simulink model "obsmod_mdl"  (R2021b)
settings: Solver=ode1  StartTime=0.0  StopTime=10  FixedStep=0.001  MaxStep=0.25  MinStep=0.01  RelTol=1e-3  EnableMultiTasking=on
values from neighbouring files (symbols this model uses):
  A = [0 1; 0 0]    [pendulum_data.m]
  Am = A+B*Lx    [obsmod_data.m]    (also in outmod_data.m; outmodc_data.m; stmod_data.m = A+B*F)
  B = [0;1]    [pendulum_data.m]
  Bm = B*-inv(Cm*inv(Am)*B)    [obsmod_data.m]    (also in outmod_data.m; outmodc_data.m; stmod_data.m = B*G)
  C = C([1,3],:)    [comp_data.m]    (also in pendulum_data.m = [1 1])
  G = -inv(C*inv(A+B*F)*B)    [obsint_data.m]    (also in stmod_data.m = -inv(H*inv(A+B*F)*B))
  L = -inv(S*B)*(S*Am-Phi*S)    [stmod_data.m]
  rho = 1    [comp_data.m]    (also in obsint_data.m; obsmod_data.m; outmod_data.m; outmodc_data.m)
  S = rpp(A,B,psm)    [obsint_data.m]    (also in stint_data.m = rpp(A,B,sp); stmod_data.m = inv(S*B)*S; streg_data.m = rpp(A,B,sp))
  x0 = zeros(1,n)    [comp_data.m]    (also in obsint_data.m; obsmod_data.m; outmod_data.m; outmodc_data.m)
  z0 = zeros(1,n)    [obsint_data.m]    (also in obsmod_data.m; pendulum_data.m)
undefined symbols (not defined in the file or in its folder): F, Lr, Lx, m, n, P
settings Model: Creator=w.schwamm  LastModifiedBy=w.schwamm
settings SolverCC: AlgebraicLoopSolver=TrustRegion
settings DataIOCC: SaveOutput=off  SaveTime=off  ReturnWorkspaceOutputs=off  StateSaveName=x  TimeSaveName=t  OutputSaveName=y
settings OptimizationCC: LifeSpan=inf
settings DebuggingCC: SFUnexpectedBacktrackingDiag=warning  SFNoUnconditionalDefaultTransitionDiag=warning  SFMachineParentedDataDiag=warning  ArithmeticOperatorsInVariantConditions=warning
settings SFSimCC: SimUseLocalCustomCode=off  CustomCodeUndefinedFunction=UseInterfaceOnly
settings RTWCC: RTWUseLocalCustomCode=off
settings CodeAppCC: StateflowObjectComments=on
settings GRTTargetCC: TargetLangStandard=C89/C90 (ANSI)
settings ConfigComp: CovMetricSettings=dw  CovSaveCumulativeToWorkspaceVar=on  CovSaveSingleToWorkspaceVar=on  CovExternalEMLEnable=off

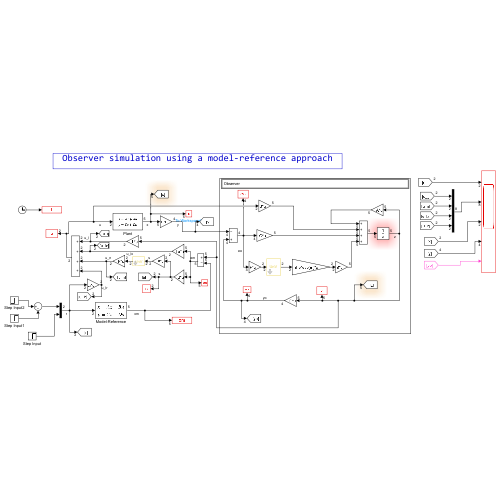
[thumbnail: Simulink's stored preview of the top-level diagram]
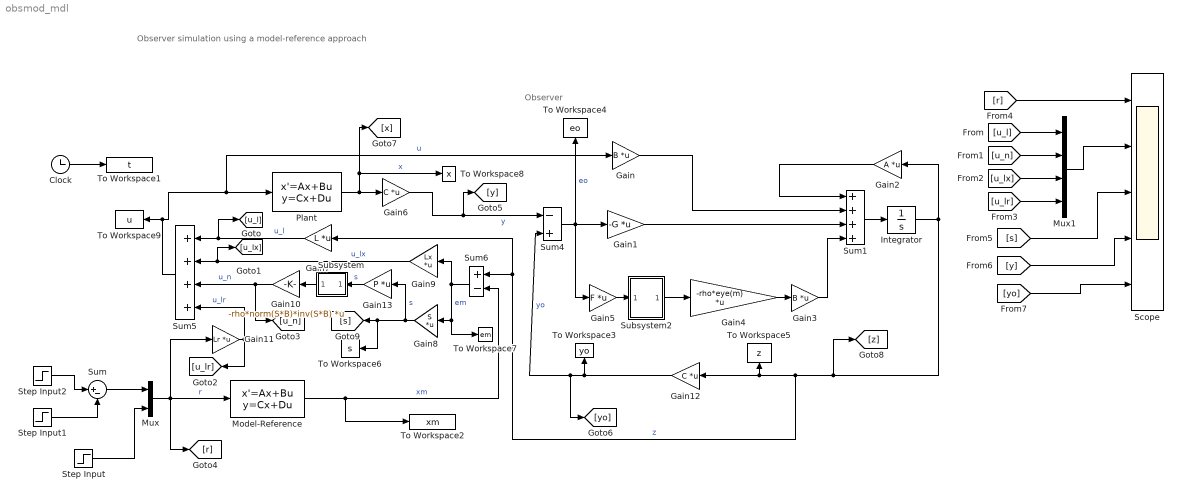
== system obsmod_mdl ==
  note: Observer
  note: Observer simulation using a model-reference approach
  Clock : Clock
  Gain : Gain  Gain=B  Multiplication=Matrix(K*u)
  Gain1 : Gain  Gain=-G  Multiplication=Matrix(K*u)
  Gain10 : Gain  Gain=-rho*norm(S*B)*inv(S*B)  Multiplication=Matrix(K*u)
  Gain11 : Gain  Gain=Lr  Multiplication=Matrix(K*u)
  Gain12 : Gain  Gain=C  Multiplication=Matrix(K*u)
  Gain13 : Gain  Gain=P  Multiplication=Matrix(K*u)
  Gain2 : Gain  Gain=A  Multiplication=Matrix(K*u)
  Gain3 : Gain  Gain=B  Multiplication=Matrix(K*u)
  Gain4 : Gain  Gain=-rho*eye(m)  Multiplication=Matrix(K*u)
  Gain5 : Gain  Gain=F  Multiplication=Matrix(K*u)
  Gain6 : Gain  Gain=C  Multiplication=Matrix(K*u)
  Gain7 : Gain  Gain=L  Multiplication=Matrix(K*u)
  Gain8 : Gain  Gain=S  Multiplication=Matrix(K*u)
  Gain9 : Gain  Gain=Lx  Multiplication=Matrix(K*u)
  Integrator : Integrator  InitialCondition=z0
  Model-Reference : StateSpace  A=Am  B=Bm  C=eye(n)  D=zeros(n,m)  InitialCondition=0
  Mux : Mux  Inputs=2
  Mux1 : Mux
  Plant : StateSpace  A=A  B=B  C=eye(n)  D=zeros(n,m)  InitialCondition=x0
  Scope : Scope  NumInputPorts=5
  Step Input : Step  Time=0  After=0*0.5  SampleTime=0
  Step Input1 : Step  Time=80  After=0  SampleTime=0
  Step Input2 : Step  Time=0  After=1*0.25  SampleTime=0
  Subsystem : Subsystem  mask{delta=0.001}
      mask prompts: delta "Unit vector delta:"
      mask Display: disp('UnV')
  Subsystem2 : Subsystem  mask{delta=0.01}
      mask prompts: delta "Unit vector delta:"
      mask Display: disp('UnV')
  Sum : Sum  Inputs=|+-
  Sum1 : Sum  Inputs=++++  InputSameDT=on  SaturateOnIntegerOverflow=on  OutDataTypeStr=Inherit: Same as first input
  Sum4 : Sum  Inputs=-+  InputSameDT=on  SaturateOnIntegerOverflow=on  OutDataTypeStr=Inherit: Same as first input
  Sum5 : Sum  Inputs=++++  InputSameDT=on  SaturateOnIntegerOverflow=on  OutDataTypeStr=Inherit: Same as first input
  Sum6 : Sum  Inputs=+-  InputSameDT=on  SaturateOnIntegerOverflow=on  OutDataTypeStr=Inherit: Same as first input
  To Workspace1 : ToWorkspace  VariableName=t  SaveFormat=Timeseries  SampleTime=-1
      settings: MaxDataPoints=1000000
  To Workspace2 : ToWorkspace  VariableName=xm  SaveFormat=Timeseries  SampleTime=-1
      settings: MaxDataPoints=1000000
  To Workspace3 : ToWorkspace  VariableName=yo  SaveFormat=Timeseries  SampleTime=-1
      settings: MaxDataPoints=1000000
  To Workspace4 : ToWorkspace  VariableName=eo  SaveFormat=Timeseries  SampleTime=-1
      settings: MaxDataPoints=1000000
  To Workspace5 : ToWorkspace  VariableName=z  SaveFormat=Timeseries  SampleTime=-1
      settings: MaxDataPoints=1000000
  To Workspace6 : ToWorkspace  VariableName=s  SaveFormat=Timeseries  SampleTime=-1
      settings: MaxDataPoints=1000000
  To Workspace7 : ToWorkspace  VariableName=em  SaveFormat=Timeseries  SampleTime=-1
      settings: MaxDataPoints=1000000
  To Workspace8 : ToWorkspace  VariableName=x  SaveFormat=Timeseries  SampleTime=-1
      settings: MaxDataPoints=1000000
  To Workspace9 : ToWorkspace  VariableName=u  SaveFormat=Timeseries  SampleTime=-1
      settings: MaxDataPoints=1000000
  wires:
  Sum6/1 -> Gain9/1, To Workspace7/1, Gain8/1  "em"
  Plant/1 -> Gain6/1, [x], To Workspace8/1  "x"
  Model-Reference/1 -> To Workspace2/1, Sum6/2  "xm"
  Gain7/1 -> [u_l], Sum5/1  "u_l"
  Integrator/1 -> Gain2/1, [z], Sum6/1, Gain7/1, Gain12/1, To Workspace5/1  "z"
  Gain9/1 -> [u_lx], Sum5/2  "u_lx"
  Gain10/1 -> [u_n], Sum5/3  "u_n"
  Gain11/1 -> Sum5/4, [u_lr]  "u_lr"
  Sum5/1 -> Gain/1, Plant/1, To Workspace9/1  "u"
  Gain6/1 -> [y], Sum4/1  "y"
  Gain8/1 -> Gain13/1, To Workspace6/1, [s]  "s"
  Gain12/1 -> [yo], Sum4/2, To Workspace3/1  "yo"
  Sum4/1 -> Gain1/1, To Workspace4/1, Gain5/1  "eo"
  Gain4/1 -> Gain3/1
  Gain5/1 -> Subsystem2/1(In1)
  Gain3/1 -> Sum1/4
  Gain1/1 -> Sum1/3
  Gain/1 -> Sum1/2
  Gain2/1 -> Sum1/1
  Sum1/1 -> Integrator/1
  Clock/1 -> To Workspace1/1
  Step Input/1 -> Mux/2
  Subsystem/1(Out1) -> Gain10/1
  Subsystem2/1(Out1) -> Gain4/1
  Mux/1 -> [r], Gain11/1, Model-Reference/1  "r"
  Sum/1 -> Mux/1
  Step Input1/1 -> Sum/2
  Step Input2/1 -> Sum/1
  [u_l] -> Mux1/1
  [u_n] -> Mux1/2
  [u_lx] -> Mux1/3
  [u_lr] -> Mux1/4
  [r] -> Scope/1
  Mux1/1 -> Scope/2
  [s] -> Scope/3
  [y] -> Scope/4
  [yo] -> Scope/5
  Gain13/1 -> Subsystem/1(In1)  "s"

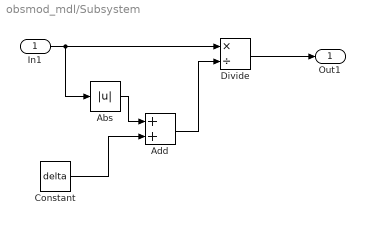
== system obsmod_mdl/Subsystem ==
  In1 : Inport
  Abs : Abs
  Add : Sum
  Constant : Constant  Value=delta  SampleTime=-1
  Divide : Product  Inputs=*/
  Out1 : Outport
  wires:
  In1/1 -> Abs/1, Divide/1
  Divide/1 -> Out1/1
  Abs/1 -> Add/1
  Add/1 -> Divide/2
  Constant/1 -> Add/2

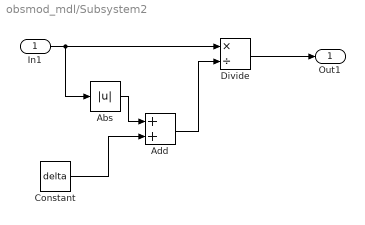
== system obsmod_mdl/Subsystem2 ==
  In1 : Inport
  Abs : Abs
  Add : Sum
  Constant : Constant  Value=delta  SampleTime=-1
  Divide : Product  Inputs=*/
  Out1 : Outport
  wires:
  In1/1 -> Abs/1, Divide/1
  Divide/1 -> Out1/1
  Abs/1 -> Add/1
  Add/1 -> Divide/2
  Constant/1 -> Add/2
